simulink model "torq_follower_base"  (R2024b)
settings: Solver=VariableStepAuto  StartTime=0.0  StopTime=10.0  RelTol=1e-3
settings Model: Creator=lukec  LastModifiedBy=lukec
settings SolverCC: ZeroCrossControl=DisableAll

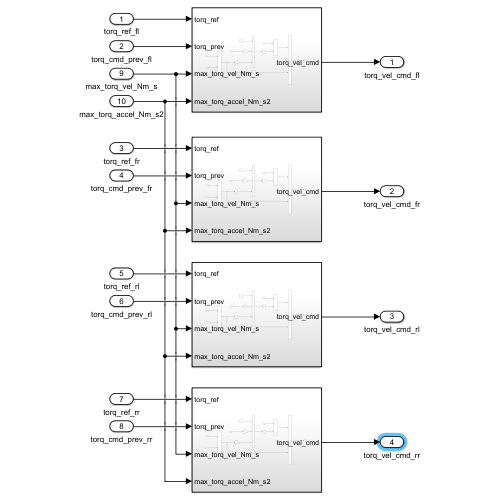
[thumbnail: Simulink's stored preview of the top-level diagram]
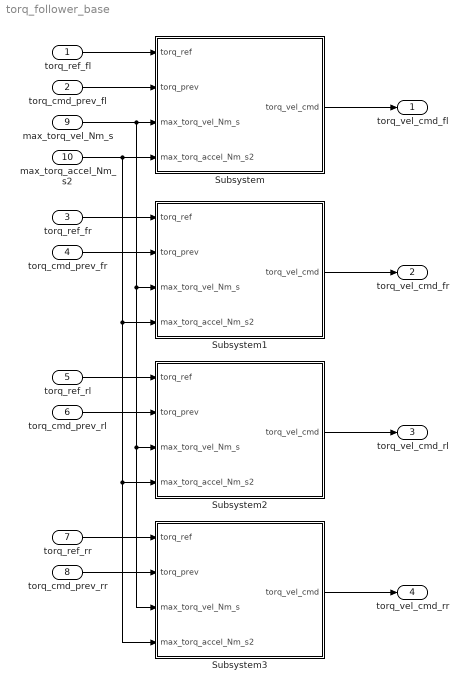
== system torq_follower_base ==
  torq_ref_fl : Inport
  torq_cmd_prev_fl : Inport  Port=2
  torq_ref_fr : Inport  Port=3
  torq_cmd_prev_fr : Inport  Port=4
  torq_ref_rl : Inport  Port=5
  torq_cmd_prev_rl : Inport  Port=6
  torq_ref_rr : Inport  Port=7
  torq_cmd_prev_rr : Inport  Port=8
  max_torq_vel_Nm_s : Inport  Port=9
  max_torq_accel_Nm_s2 : Inport  Port=10
  Subsystem : Subsystem
  Subsystem1 : Subsystem
  Subsystem2 : Subsystem
  Subsystem3 : Subsystem
  torq_vel_cmd_fl : Outport
  torq_vel_cmd_fr : Outport  Port=2
  torq_vel_cmd_rl : Outport  Port=3
  torq_vel_cmd_rr : Outport  Port=4
  wires:
  torq_ref_fl/1 -> Subsystem/1(torq_ref)
  torq_cmd_prev_fl/1 -> Subsystem/2(torq_prev)
  Subsystem/1(torq_vel_cmd) -> torq_vel_cmd_fl/1
  torq_ref_fr/1 -> Subsystem1/1(torq_ref)
  Subsystem1/1(torq_vel_cmd) -> torq_vel_cmd_fr/1
  torq_cmd_prev_fr/1 -> Subsystem1/2(torq_prev)
  torq_ref_rl/1 -> Subsystem2/1(torq_ref)
  Subsystem2/1(torq_vel_cmd) -> torq_vel_cmd_rl/1
  torq_cmd_prev_rl/1 -> Subsystem2/2(torq_prev)
  Subsystem3/1(torq_vel_cmd) -> torq_vel_cmd_rr/1
  torq_ref_rr/1 -> Subsystem3/1(torq_ref)
  torq_cmd_prev_rr/1 -> Subsystem3/2(torq_prev)
  max_torq_vel_Nm_s/1 -> Subsystem3/3(max_torq_vel_Nm_s), Subsystem2/3(max_torq_vel_Nm_s), Subsystem1/3(max_torq_vel_Nm_s), Subsystem/3(max_torq_vel_Nm_s)
  max_torq_accel_Nm_s2/1 -> Subsystem/4(max_torq_accel_Nm_s2), Subsystem1/4(max_torq_accel_Nm_s2), Subsystem2/4(max_torq_accel_Nm_s2), Subsystem3/4(max_torq_accel_Nm_s2)

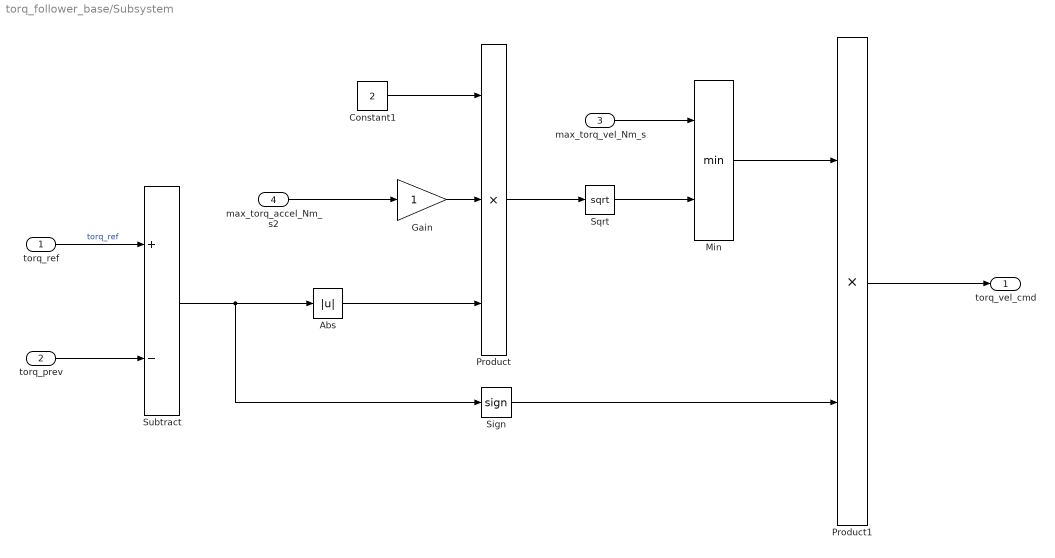
== system torq_follower_base/Subsystem ==
  torq_ref : Inport
  torq_prev : Inport  Port=2
  max_torq_vel_Nm_s : Inport  Port=3
  max_torq_accel_Nm_s2 : Inport  Port=4
  Abs : Abs  SaturateOnIntegerOverflow=off
  Constant1 : Constant  Value=2
  Gain : Gain
  Min : MinMax  Inputs=2
  Product : Product  Inputs=3
  Product1 : Product
  Sign : Signum
  Sqrt : Sqrt
  Subtract : Sum  Inputs=+-
  torq_vel_cmd : Outport
  wires:
  torq_ref/1 -> Subtract/1  "torq_ref"
  max_torq_accel_Nm_s2/1 -> Gain/1
  Product/1 -> Sqrt/1
  Sign/1 -> Product1/2
  Min/1 -> Product1/1
  max_torq_vel_Nm_s/1 -> Min/1
  Constant1/1 -> Product/1
  Abs/1 -> Product/3
  Subtract/1 -> Sign/1, Abs/1
  Sqrt/1 -> Min/2
  Gain/1 -> Product/2
  torq_prev/1 -> Subtract/2
  Product1/1 -> torq_vel_cmd/1

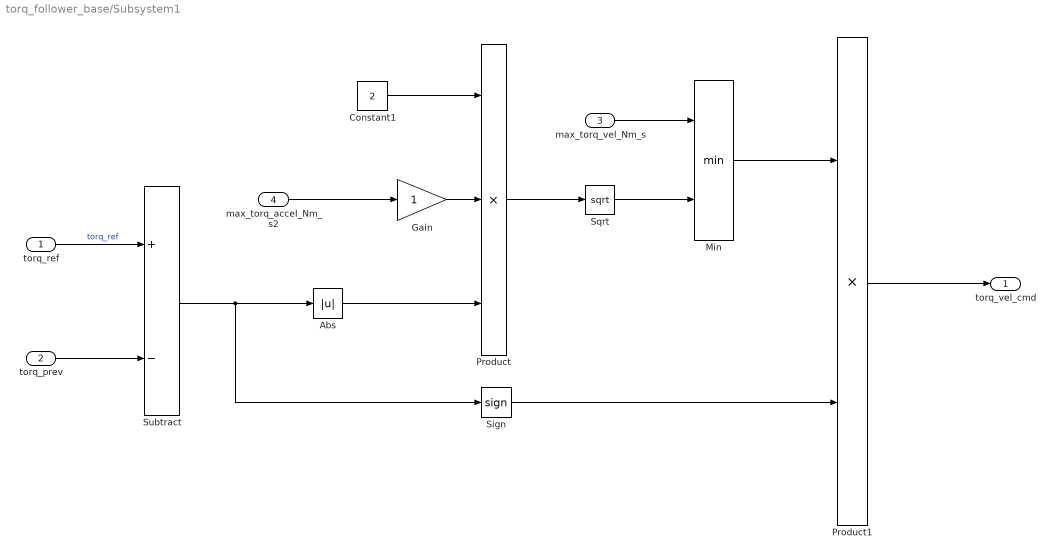
== system torq_follower_base/Subsystem1 ==
  torq_ref : Inport
  torq_prev : Inport  Port=2
  max_torq_vel_Nm_s : Inport  Port=3
  max_torq_accel_Nm_s2 : Inport  Port=4
  Abs : Abs  SaturateOnIntegerOverflow=off
  Constant1 : Constant  Value=2
  Gain : Gain
  Min : MinMax  Inputs=2
  Product : Product  Inputs=3
  Product1 : Product
  Sign : Signum
  Sqrt : Sqrt
  Subtract : Sum  Inputs=+-
  torq_vel_cmd : Outport
  wires:
  Product1/1 -> torq_vel_cmd/1
  torq_prev/1 -> Subtract/2
  Gain/1 -> Product/2
  Sqrt/1 -> Min/2
  Subtract/1 -> Abs/1, Sign/1
  Abs/1 -> Product/3
  Constant1/1 -> Product/1
  max_torq_vel_Nm_s/1 -> Min/1
  Min/1 -> Product1/1
  Sign/1 -> Product1/2
  Product/1 -> Sqrt/1
  max_torq_accel_Nm_s2/1 -> Gain/1
  torq_ref/1 -> Subtract/1  "torq_ref"

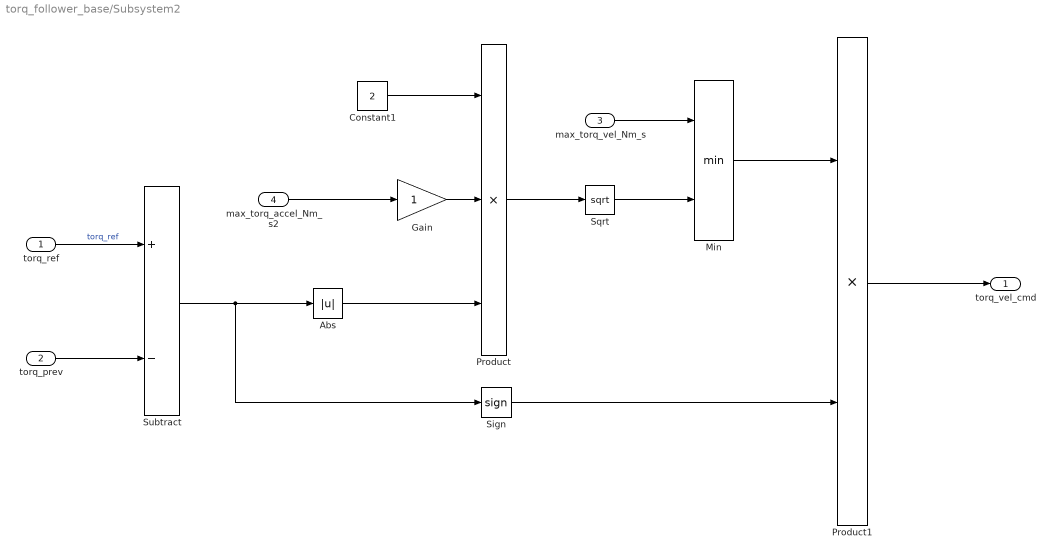
== system torq_follower_base/Subsystem2 ==
  torq_ref : Inport
  torq_prev : Inport  Port=2
  max_torq_vel_Nm_s : Inport  Port=3
  max_torq_accel_Nm_s2 : Inport  Port=4
  Abs : Abs  SaturateOnIntegerOverflow=off
  Constant1 : Constant  Value=2
  Gain : Gain
  Min : MinMax  Inputs=2
  Product : Product  Inputs=3
  Product1 : Product
  Sign : Signum
  Sqrt : Sqrt
  Subtract : Sum  Inputs=+-
  torq_vel_cmd : Outport
  wires:
  torq_ref/1 -> Subtract/1  "torq_ref"
  max_torq_accel_Nm_s2/1 -> Gain/1
  Product/1 -> Sqrt/1
  Sign/1 -> Product1/2
  Min/1 -> Product1/1
  max_torq_vel_Nm_s/1 -> Min/1
  Constant1/1 -> Product/1
  Abs/1 -> Product/3
  Subtract/1 -> Sign/1, Abs/1
  Sqrt/1 -> Min/2
  Gain/1 -> Product/2
  torq_prev/1 -> Subtract/2
  Product1/1 -> torq_vel_cmd/1

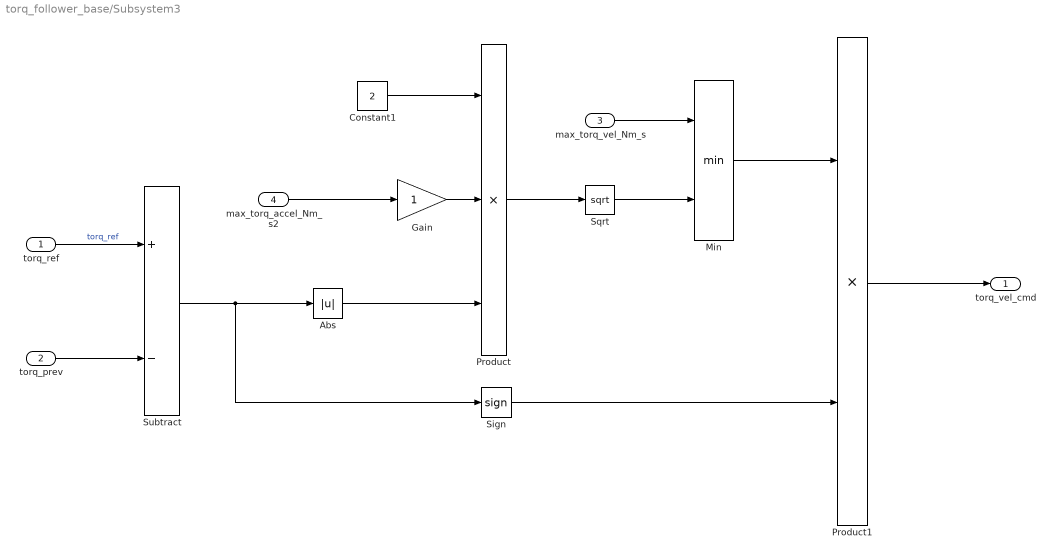
== system torq_follower_base/Subsystem3 ==
  torq_ref : Inport
  torq_prev : Inport  Port=2
  max_torq_vel_Nm_s : Inport  Port=3
  max_torq_accel_Nm_s2 : Inport  Port=4
  Abs : Abs  SaturateOnIntegerOverflow=off
  Constant1 : Constant  Value=2
  Gain : Gain
  Min : MinMax  Inputs=2
  Product : Product  Inputs=3
  Product1 : Product
  Sign : Signum
  Sqrt : Sqrt
  Subtract : Sum  Inputs=+-
  torq_vel_cmd : Outport
  wires:
  Product1/1 -> torq_vel_cmd/1
  torq_prev/1 -> Subtract/2
  Gain/1 -> Product/2
  Sqrt/1 -> Min/2
  Subtract/1 -> Abs/1, Sign/1
  Abs/1 -> Product/3
  Constant1/1 -> Product/1
  max_torq_vel_Nm_s/1 -> Min/1
  Min/1 -> Product1/1
  Sign/1 -> Product1/2
  Product/1 -> Sqrt/1
  max_torq_accel_Nm_s2/1 -> Gain/1
  torq_ref/1 -> Subtract/1  "torq_ref"
